simulink subsystem "vector_sin_controller"  (R2023a)
settings: Solver=VariableStepAuto  StartTime=0.0  StopTime=10.0  RelTol=1e-3
undefined symbols (not defined in the file): motor_poly_count, SG_angular_accel_limit, SG_smoother_gain
settings Model: Creator=motya  LastModifiedBy=motya

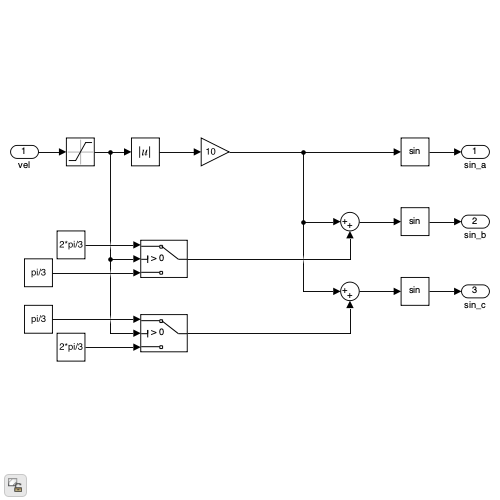
[thumbnail: Simulink's stored preview of the top-level diagram]
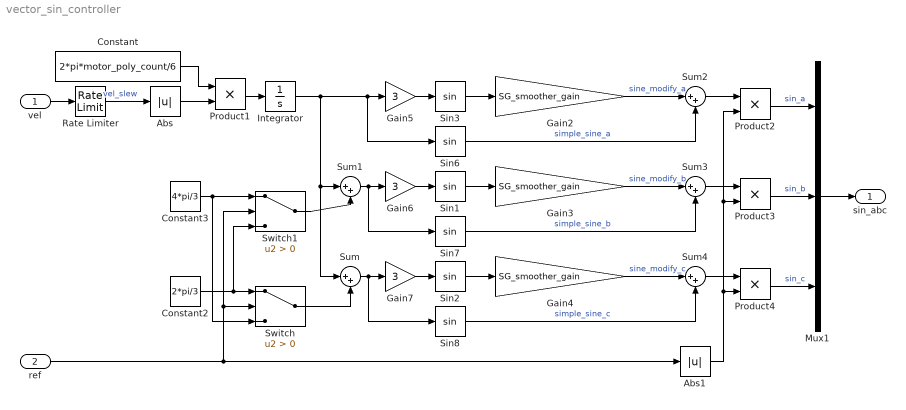
== system vector_sin_controller ==
  vel : Inport
  ref : Inport  Port=2
  Abs : Abs  SaturateOnIntegerOverflow=off
  Abs1 : Abs  SaturateOnIntegerOverflow=off
  Constant : Constant  Value=2*pi*motor_poly_count/6
  Constant2 : Constant  Value=2*pi/3
  Constant3 : Constant  Value=4*pi/3
  Gain2 : Gain  Gain=SG_smoother_gain
  Gain3 : Gain  Gain=SG_smoother_gain
  Gain4 : Gain  Gain=SG_smoother_gain
  Gain5 : Gain  Gain=3
  Gain6 : Gain  Gain=3
  Gain7 : Gain  Gain=3
  Integrator : Integrator
  Mux1 : Mux  Inputs=3
  Product{1..4} (4 alike) : Product
  Rate Limiter : RateLimiter  RisingSlewLimit=SG_angular_accel_limit  FallingSlewLimit=-SG_angular_accel_limit  SampleTimeMode=inherited
  Sin{1..3,6..8} (6 alike) : Trigonometry
  Sum{,1..4} (5 alike) : Sum  Inputs=|++
  Switch : Switch  Criteria=u2 > Threshold  SaturateOnIntegerOverflow=off  InputSameDT=off
  Switch1 : Switch  Criteria=u2 > Threshold  SaturateOnIntegerOverflow=off  InputSameDT=off
  sin_abc : Outport
  wires:
  Sum/1 -> Gain7/1, Sin8/1
  Sum1/1 -> Gain6/1, Sin7/1
  Switch/1 -> Sum/2
  Constant3/1 -> Switch1/1, Switch/3
  Constant2/1 -> Switch/1, Switch1/3
  Abs/1 -> Product1/2
  Product1/1 -> Integrator/1
  Sum2/1 -> Product2/1
  Sum3/1 -> Product3/1
  Sum4/1 -> Product4/1
  Sin3/1 -> Gain2/1
  Sin1/1 -> Gain3/1
  Sin2/1 -> Gain4/1
  Product2/1 -> Mux1/1  "sin_a"
  Product3/1 -> Mux1/2  "sin_b"
  Product4/1 -> Mux1/3  "sin_c"
  vel/1 -> Rate Limiter/1
  Constant/1 -> Product1/1
  Integrator/1 -> Sum1/1, Sum/1, Gain5/1, Sin6/1
  Gain5/1 -> Sin3/1
  Gain6/1 -> Sin1/1
  Gain7/1 -> Sin2/1
  Gain4/1 -> Sum4/1  "sine_modify_c"
  Sin8/1 -> Sum4/2  "simple_sine_c"
  Sin7/1 -> Sum3/2  "simple_sine_b"
  Sin6/1 -> Sum2/2  "simple_sine_a"
  Gain3/1 -> Sum3/1  "sine_modify_b"
  Gain2/1 -> Sum2/1  "sine_modify_a"
  ref/1 -> Abs1/1, Switch1/2, Switch/2
  Switch1/1 -> Sum1/2
  Abs1/1 -> Product4/2, Product3/2, Product2/2
  Mux1/1 -> sin_abc/1
  Rate Limiter/1 -> Abs/1  "vel_slew"
